simulink model "idhp_model_heart_realtime_synReduit"  (R2014a)
settings: Solver=FixedStepDiscrete  StartTime=0.0  StopTime=100  FixedStep=0.01  RelTol=1e-3
values from neighbouring files (symbols this model uses):
  Atr_refrD = 50    [const.m]
  AV_alpha = 150    [const.m]
  AV_anteDMin = 50    [const.m]
  AV_beta = 250    [const.m]
  AV_delta = 10    [const.m]
  AV_k4 = 0.03    [const.m]
  AV_refrDMin = 50    [const.m]
  AV_retroDMin = 100    [const.m]
  AV_tauC = 100    [const.m]
  AV_theta = 10    [const.m]
  AV_tr = 500    [const.m]
  AV_Vr = -90    [const.m]
  AV_Vt = -40    [const.m]
  PM_TAVI = 150    [const.m]
  PM_TLRI = 1000    [const.m]
  PM_TPVAB = 50    [const.m]
  PM_TPVARP = 250    [const.m]
  PM_TURI = 500    [const.m]
  PM_TVRP = 320    [const.m]
  RA_anteD = 30    [const.m]
  RA_retroD = 30    [const.m]
  RV_anteD = 50    [const.m]
  RV_retroD = 50    [const.m]
  SA_d = 850    [const.m]
  SA_dV = 50    [const.m]
  SA_ectopD = 10400    [const.m]
  SA_ectopdV = 50    [const.m]
  SA_noiseD = 1.0E+6    (= 1000000)    [const.m]
  VRG_d = 3000    [const.m]
  VRG_ectopD = 30450    [const.m]
  VRG_noiseD = 1.0E+6    (= 1000000)    [const.m]
  Vtr_refrD = 200    [const.m]
libraries: simulink x4
settings Model: Creator=alexandru  LastModifiedBy=barbot
settings DataIOCC: LimitDataPoints=off  SaveOutput=off  SignalLogging=off  DSMLogging=off  SaveTime=off
settings HardwareCC: TargetBitPerLong=64  TargetBitPerPointer=64  TargetLongLongMode=on  TargetIntDivRoundTo=Zero  TargetEndianess=LittleEndian  TargetWordSize=64  TargetHWDeviceType=MATLAB Host  ProdEqTarget=off
settings RTWCC: SystemTargetFile=rsim.tlc  GenCodeOnly=on  PackageGeneratedCodeAndArtifacts=on  PackageName=idhp_model_heart_realtime  TemplateMakefile=rsim_default_tmf  Description=Rapid Simulation Target  ProcessScript=rsim_make_rtw_hook
settings RSimTargetCC: ERTMultiwordTypeDef=System defined  ERTMultiwordLength=256  EnableShiftOperators=on

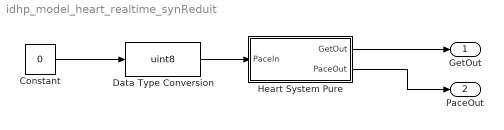
== system idhp_model_heart_realtime_synReduit ==
  Constant : Constant  Value=0
  Data Type Conversion : DataTypeConversion  OutDataTypeStr=uint8
  Heart System Pure : Subsystem
  GetOut : Outport
  PaceOut : Outport  Port=2
  wires:
  Data Type Conversion/1 -> Heart System Pure/1(PaceIn)
  Heart System Pure/1(GetOut) -> GetOut/1
  Heart System Pure/2(PaceOut) -> PaceOut/1
  Constant/1 -> Data Type Conversion/1

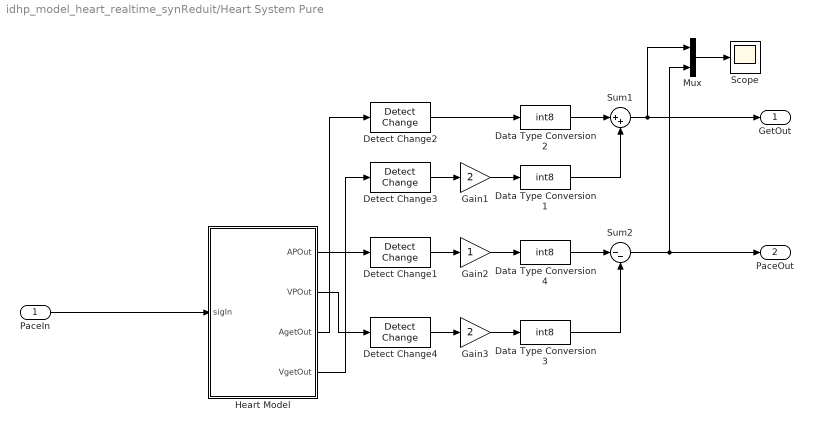
== system idhp_model_heart_realtime_synReduit/Heart System Pure ==
  PaceIn : Inport
  Data Type Conversion{1..4} (4 alike) : DataTypeConversion  OutDataTypeStr=int8
  Detect Change1 : simulink/Logic and Bit Operations/Detect Change  vinit=0  InputProcessing=Inherited  OutDataTypeStr=uint8
  Detect Change2 : simulink/Logic and Bit Operations/Detect Change  vinit=0  InputProcessing=Inherited  OutDataTypeStr=uint8
  Detect Change3 : simulink/Logic and Bit Operations/Detect Change  vinit=0  InputProcessing=Inherited  OutDataTypeStr=boolean
  Detect Change4 : simulink/Logic and Bit Operations/Detect Change  vinit=0  InputProcessing=Inherited  OutDataTypeStr=uint8
  Gain1 : Gain  Gain=2
  Gain2 : Gain
  Gain3 : Gain  Gain=2
  Heart Model : Stateflow chart  Priority=1  TreatAsAtomicUnit=on
  Mux : Mux  Inputs=2
  Scope : Scope
  Sum1 : Sum  Inputs=|++
  Sum2 : Sum  Inputs=|--
  GetOut : Outport
  PaceOut : Outport  Port=2
  wires:
  Detect Change3/1 -> Gain1/1
  Gain1/1 -> Data Type Conversion1/1
  Sum1/1 -> Mux/1, GetOut/1
  Data Type Conversion1/1 -> Sum1/2
  Detect Change2/1 -> Data Type Conversion2/1
  Data Type Conversion2/1 -> Sum1/1
  Heart Model/1(APOut) -> Detect Change1/1
  Heart Model/2(VPOut) -> Detect Change4/1
  Detect Change4/1 -> Gain3/1
  Gain3/1 -> Data Type Conversion3/1
  Data Type Conversion3/1 -> Sum2/2
  Data Type Conversion4/1 -> Sum2/1
  Sum2/1 -> PaceOut/1, Mux/2
  PaceIn/1 -> Heart Model/1(sigIn)
  Heart Model/4(VgetOut) -> Detect Change3/1
  Heart Model/3(AgetOut) -> Detect Change2/1
  Mux/1 -> Scope/1
  Detect Change1/1 -> Gain2/1
  Gain2/1 -> Data Type Conversion4/1

== stateflow chart idhp_model_heart_realtime_synReduit/Heart System Pure/Heart Model ==
  state Heart
    state RE_AVJOut [parallel]
      settings: executionOrder=1
      state Empty
      state Ante
      state Retro
      (default) -> Heart.RE_AVJOut.Empty
      Heart.RE_AVJOut.Ante -> Heart.RE_AVJOut.Empty : after(AV_anteDMin,msec)
          | {send(anteAVJ,RVConductor);}
      Heart.RE_AVJOut.Empty -> Heart.RE_AVJOut.Ante [order 1] : AVJAnteExit
      Heart.RE_AVJOut.Retro -> Heart.RE_AVJOut.Empty : after(AV_retroDMin,msec)
          | {send(retroAVJ,RAConductor);}
      Heart.RE_AVJOut.Empty -> Heart.RE_AVJOut.Retro [order 2] : AVJRetroExit
    state RE_RAConductor [parallel]
      settings: executionOrder=3
      state Empty
      state Ante
      state Retro
      (default) -> Heart.RE_RAConductor.Empty
      Heart.RE_RAConductor.Empty -> Heart.RE_RAConductor.Ante [order 1] : arg
      Heart.RE_RAConductor.Ante -> Heart.RE_RAConductor.Empty [order 1] : retroAVJ
      Heart.RE_RAConductor.Empty -> Heart.RE_RAConductor.Retro [order 2] : retroAVJ
      Heart.RE_RAConductor.Retro -> Heart.RE_RAConductor.Empty [order 1] : arg
      Heart.RE_RAConductor.Retro -> Heart.RE_RAConductor.Empty [order 2] : after(RA_retroD,msec)
          | {send(AtrRetroReached,...
          | Atrium);}
      Heart.RE_RAConductor.Ante -> Heart.RE_RAConductor.Empty [order 2] : after(RA_anteD,msec)
          | {send(AVJAnteReached,AVJ);}
    state RE_RVConductor [parallel]
      settings: executionOrder=2
      state Empty
      state Ante
      state Retro
      (default) -> Heart.RE_RVConductor.Empty
      Heart.RE_RVConductor.Empty -> Heart.RE_RVConductor.Ante [order 1] : anteAVJ
      Heart.RE_RVConductor.Empty -> Heart.RE_RVConductor.Retro [order 2] : vrg
      Heart.RE_RVConductor.Ante -> Heart.RE_RVConductor.Empty [order 1] : vrg
      Heart.RE_RVConductor.Ante -> Heart.RE_RVConductor.Empty [order 2] : after(RV_anteD,msec)
          | {send(VtrAnteReached,...
          | Ventricle);}
      Heart.RE_RVConductor.Retro -> Heart.RE_RVConductor.Empty [order 1] : anteAVJ
      Heart.RE_RVConductor.Retro -> Heart.RE_RVConductor.Empty [order 2] : after(RV_retroD,msec)
          | {send(AVJRetroReached,...
          | AVJ);}
    state RE_SANode [parallel]
      settings: executionOrder=4
      state Wait4ABeat
      state Wait4ASynch
      (default) -> Wait4ABeat
      Wait4ABeat -> Wait4ASynch [order 2] : after(SA_d, msec)
          | {send(Abeat,Atrium);
          | }
      Wait4ABeat -> Wait4ABeat [order 1] : NextAtrBeat
      Wait4ASynch -> Wait4ABeat : NextAtrBeat
    state RE_VRG [parallel]
      settings: executionOrder=7
      state Wait4VBeat
      state Wait4VSynch
      (default) -> Wait4VBeat
      Wait4VBeat -> Wait4VSynch [order 2] : after(VRG_d, msec)
          | {send(Vbeat,Ventricle);}
      Wait4VSynch -> Wait4VBeat : NextVtrBeat
      Wait4VBeat -> Wait4VBeat [order 1] : NextVtrBeat
    state RE_AVJ [parallel]
      settings: executionOrder=10
      state Recovery
      state Refractory
      (default) -> Recovery
      Recovery -> Heart.RE_AVJ.Refractory [order 1] : AVJAnteReached{send(AVJAnteExit,AVJOut);
          | }
      Heart.RE_AVJ.Refractory -> Recovery : after(258,msec)
      Recovery -> Heart.RE_AVJ.Refractory [order 3] : AVJRetroReached{
          | send(AVJRetroExit,AVJOut);
          | }
      Recovery -> Heart.RE_AVJ.Refractory [order 2] : after(Reduce_TimeToDep,msec){
          | }
    state RE_Ventricle [parallel]
      settings: executionOrder=5
      state Excitable
      state Refractory
      state Vsense
      (default) -> Heart.RE_Ventricle.Refractory
      Heart.RE_Ventricle.Refractory -> Heart.RE_Ventricle.Excitable : after(Vtr_refrD,msec)
      Heart.RE_Ventricle.Excitable -> Heart.RE_Ventricle.Refractory [order 1] : VtrAnteReached{
          | send(Vget,VRP);
          | send(NextVtrBeat,VRG);
          | }
      Heart.RE_Ventricle.Excitable -> Vsense [order 3] : Vbeat{
          | send(Vget,VRP);
          | }
      Vsense -> Heart.RE_Ventricle.Refractory : {
          | send(NextVtrBeat,VRG);
          | send(vrg,RVConductor);
          | }
      Heart.RE_Ventricle.Excitable -> Vsense [order 2] : VP
    state RE_Atrium [parallel]
      settings: executionOrder=6
      state Excitable
      state Refractory
      state Asense
      (default) -> Heart.RE_Atrium.Refractory
      Heart.RE_Atrium.Refractory -> Heart.RE_Atrium.Excitable : after(Atr_refrD,msec)
      Heart.RE_Atrium.Excitable -> Heart.RE_Atrium.Refractory [order 1] : AtrRetroReached{
          | send(Aget,PVARP);
          | send(NextAtrBeat,SANode);
          | }
      Asense -> Heart.RE_Atrium.Refractory : {
          | send(arg,RAConductor);
          | send(NextAtrBeat,SANode);
          | }
      Heart.RE_Atrium.Excitable -> Asense [order 2] : APace
      Heart.RE_Atrium.Excitable -> Asense [order 3] : Abeat{
          | send(Aget,PVARP);
          | }
    state RE_LRI [parallel]
      settings: executionOrder=8
      state LRI
      state LRI1
      state LRI2
      state LRI3
      LRI3 -> LRI [order 3] : after((PM_TLRI-PM_TAVI)/4,msec){
          | send(APace,Atrium);
          | send(AP,AVI);
          | }
      (default) -> LRI
      LRI1 -> LRI2 [order 1] : after((PM_TLRI-PM_TAVI)/4,msec)
      LRI -> LRI1 [order 3] : after((PM_TLRI-PM_TAVI)/4,msec)
      LRI2 -> LRI3 [order 1] : after((PM_TLRI-PM_TAVI)/4,msec)
      LRI -> LRI [order 1] : RLRI
      LRI1 -> LRI [order 3] : RLRI
      LRI1 -> LRI [order 2] : AS
      LRI2 -> LRI [order 2] : AS
    state RE_URI [parallel]
      settings: executionOrder=9
      state URI
      (default) -> URI
      URI -> URI [order 1] : RURI
      URI -> URI [order 2] : after(PM_TURI,msec){
          | send(IncrClk,AVI);
          | }
    state RE_AVI [parallel]
      settings: executionOrder=11
      state Idle0
      state AVI0
      state WaitURI
      state Idle1
      state AVI1
      WaitURI -> Idle0 [order 1] : VS{RURI;}
      AVI0 -> Idle0 [order 3] : VS{RURI;}
      Idle0 -> AVI0 [order 2] : AP{RTAVI;}
      (default) -> Idle0
      AVI0 -> WaitURI [order 2] : TAVI
      Idle0 -> AVI0 [order 3] : AS{RTAVI;}
      AVI1 -> Idle0 [order 2] : TAVI{
          | send(RLRI,LRI);
          | send(VP,VRP);
          | send(VP,PVARP);
          | send(VP,Ventricle);
          | send(RURI,URI);
          | }
      AVI1 -> Idle0 [order 1] : VS{send(RURI,URI);}
      WaitURI -> Idle0 [order 2] : IncrClk{
          | send(RLRI,LRI);
          | send(VP,VRP);
          | send(VP,PVARP);
          | send(VP,Ventricle);
          | }
      AVI0 -> AVI1 [order 1] : IncrClk
      Idle0 -> Idle1 [order 1] : IncrClk
      Idle1 -> AVI1 [order 2] : AP{send(RTAVI,TAVIcmp);}
      Idle1 -> AVI1 [order 1] : AS{send(RTAVI,TAVIcmp);}
    state VRP [parallel]
      settings: executionOrder=12
      state Idle
      (default) -> Heart.VRP.Idle
      Heart.VRP.Idle -> Heart.VRP.Idle : Vget{
          | send(RLRI, LRI);
          | send(VS, AVI);
          | }
    state PVARP [parallel]
      settings: executionOrder=13
      state Idle
      (default) -> Heart.PVARP.Idle
      Heart.PVARP.Idle -> Heart.PVARP.Idle : Aget{
          | send(AS,LRI);
          | send(AS,AVI);
          | }
    state RE_TAVIcmp [parallel]
      settings: executionOrder=14
      state q01
      state q02
      state q03
      state q0
      state q1
      q02 -> q03 [order 1] : after(PM_TAVI/4,msec)
      q01 -> q02 [order 1] : after(PM_TAVI/4,msec)
      q0 -> q01 : after(PM_TAVI/4,msec)
      q03 -> q0 [order 2] : RTAVI
      q02 -> q0 [order 2] : RTAVI
      q01 -> q0 [order 2] : RTAVI
      q03 -> q1 [order 1] : after(PM_TAVI/4,msec){send(TAVI,AVI);}
      q1 -> q0 : RTAVI
      (default) -> q1
    LRI3 -> LRI [order 2] : RLRI
    LRI2 -> LRI [order 3] : RLRI
    LRI -> LRI [order 2] : AS
    LRI3 -> LRI [order 1] : AS
  (default) -> Heart
  data: Atr_refrD parameter; AV_alpha parameter; AV_anteDMin parameter; AV_beta parameter; AV_delta parameter; AV_k4 parameter; AV_refrDMin parameter; AV_retroDMin parameter; AV_tauC parameter; AV_theta parameter; AV_tr parameter; AV_Vr parameter; AV_Vt parameter; RA_anteD parameter; RA_retroD parameter; RV_anteD parameter; RV_retroD parameter; SA_d parameter; SA_dV parameter; SA_ectopD parameter; SA_ectopdV parameter; SA_noiseD parameter; VRG_d parameter; VRG_ectopD parameter; VRG_noiseD parameter; Vtr_refrD parameter; avj_tRec local double; sigIn input uint8; clk local double; PM_TAVI parameter; PM_TLRI parameter; PM_TPVAB parameter; PM_TPVARP parameter; PM_TURI parameter; PM_TVRP parameter; recoverylast local double; avj_t4 local double; ctime local double; avj_refr local double; avj_refr_0 local double; refractorylast local double
  events: Abeat local FUNCTION_CALL_EVENT; AtrRetroReached local FUNCTION_CALL_EVENT; arg local FUNCTION_CALL_EVENT; retroAVJ local FUNCTION_CALL_EVENT; AVJAnteReached local FUNCTION_CALL_EVENT; NextAtrBeat local FUNCTION_CALL_EVENT; AVJRetroReached local FUNCTION_CALL_EVENT; anteAVJ local FUNCTION_CALL_EVENT; vrg local FUNCTION_CALL_EVENT; VtrAnteReached local FUNCTION_CALL_EVENT; AVJRetroExit local FUNCTION_CALL_EVENT; AVJAnteExit local FUNCTION_CALL_EVENT; NextVtrBeat local FUNCTION_CALL_EVENT; Vbeat local FUNCTION_CALL_EVENT; AP local EITHER_EDGE_EVENT; VP local EITHER_EDGE_EVENT; APOut output EITHER_EDGE_EVENT; VPOut output EITHER_EDGE_EVENT; AS local RISING_EDGE_EVENT; VS local RISING_EDGE_EVENT; Aget local EITHER_EDGE_EVENT; Vget local EITHER_EDGE_EVENT; Aintrinsic local EITHER_EDGE_EVENT; Anoise local EITHER_EDGE_EVENT; Aretro local EITHER_EDGE_EVENT; Vintrinsic local EITHER_EDGE_EVENT; Vnoise local EITHER_EDGE_EVENT; Vante local EITHER_EDGE_EVENT; AgetOut output EITHER_EDGE_EVENT; VgetOut output EITHER_EDGE_EVENT; APElectr local RISING_EDGE_EVENT; VPElectr local EITHER_EDGE_EVENT; IncrClk local FUNCTION_CALL_EVENT; State local FUNCTION_CALL_EVENT; Clk0 local FUNCTION_CALL_EVENT; Clk1 local FUNCTION_CALL_EVENT; a_dVSetHigh local FUNCTION_CALL_EVENT; a_dVSetLow local FUNCTION_CALL_EVENT; tr_AVJ local FUNCTION_CALL_EVENT; AVJAnteReachedHigh local FUNCTION_CALL_EVENT; TAVI local FUNCTION_CALL_EVENT; RURI local FUNCTION_CALL_EVENT; RTAVI local FUNCTION_CALL_EVENT; RLRI local FUNCTION_CALL_EVENT; APace local FUNCTION_CALL_EVENT
